simulink model "LineFollowerSim"  (R2021b)
settings: Solver=FixedStepDiscrete  StartTime=0.0  StopTime=10  FixedStep=0.1  RelTol=1e-3  EnableMultiTasking=on
libraries: arduinolib x8, arduinosensorlib x1
settings Model: ExtModeTrigDuration=2  Creator=arjun  LastModifiedBy=arjun
settings SolverCC: AlgebraicLoopSolver=TrustRegion  AutoInsertRateTranBlk=on
settings DataIOCC: LimitDataPoints=on
settings OptimizationCC: EnhancedBackFolding=on  PassReuseOutputArgsAs=Individual arguments  ZeroExternalMemoryAtStartup=off  ZeroInternalMemoryAtStartup=off  MaxStackSize=64  OptimizeBlockOrder=speed  DifferentSizesBufferReuse=on  OptimizationCustomize=off  EfficientTunableParamExpr=on
settings DebuggingCC: ParameterTunabilityLossMsg=error  AllowSymbolicDim=off  SFUnexpectedBacktrackingDiag=warning  SFNoUnconditionalDefaultTransitionDiag=warning  SFExecutionAtInitializationDiag=none  ArithmeticOperatorsInVariantConditions=warning
settings HardwareCC: ProdBitPerInt=16  ProdBitPerPointer=16  ProdBitPerSizeT=16  ProdBitPerPtrDiffT=16  ProdLargestAtomicFloat=None  ProdWordSize=8  ProdHWDeviceType=Atmel->AVR
settings SFSimCC: SimUseLocalCustomCode=off  MATLABDynamicMemAlloc=off  CustomCodeUndefinedFunction=UseInterfaceOnly
settings RTWCC: Description=Embedded Coder  SystemTargetFile=ert.tlc  HardwareBoard=Arduino Uno  TemplateMakefile=ert_default_tmf  RTWUseLocalCustomCode=off  Toolchain=Arduino AVR  BuildConfiguration=Faster Runs
settings CodeAppCC: ForceParamTrailComments=on  IgnoreCustomStorageClasses=off  OperatorAnnotations=on  SimulinkDataObjDesc=on  SFDataObjDesc=on  InsertBlockDesc=on
settings ERTTargetCC: SupportContinuousTime=on  SupportVariableSizeSignals=on  ExtModeTransport=3  ExtModeStaticAlloc=on  ExtModeStaticAllocSize=250  ExtModeMexFile=ext_xcp  ExtModeIntrfLevel=Level2 - Open
settings ConfigComp: CovMetricSettings=dw  CovSaveCumulativeToWorkspaceVar=on  CovSaveSingleToWorkspaceVar=on  CovExternalEMLEnable=off  CovSFcnEnable=off

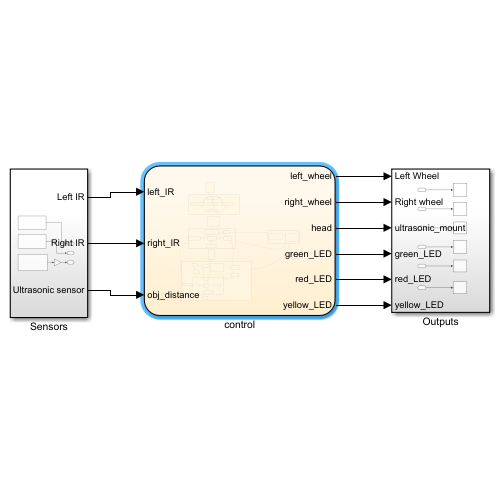
[thumbnail: Simulink's stored preview of the top-level diagram]
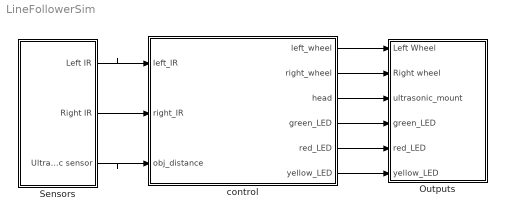
== system LineFollowerSim ==
  Outputs : Subsystem
  Sensors : Subsystem
  control : Stateflow chart  TreatAsAtomicUnit=on
  wires:
  Sensors/1(Left IR) -> control/1(left_IR)
  Sensors/2(Right IR) -> control/2(right_IR)
  Sensors/3(Ultrasonic sensor) -> control/3(obj_distance)
  control/1(left_wheel) -> Outputs/1(Left Wheel)
  control/2(right_wheel) -> Outputs/2(Right wheel)
  control/3(head) -> Outputs/3(ultrasonic_mount)
  control/4(green_LED) -> Outputs/4(green_LED)
  control/5(red_LED) -> Outputs/5(red_LED)
  control/6(yellow_LED) -> Outputs/6(yellow_LED)

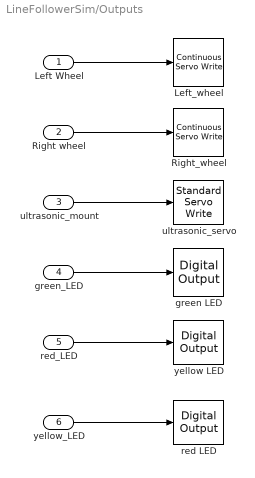
== system LineFollowerSim/Outputs ==
  Left Wheel : Inport
  Right wheel : Inport  Port=2
  ultrasonic_mount : Inport  Port=3
  green_LED : Inport  Port=4
  red_LED : Inport  Port=5
  yellow_LED : Inport  Port=6
  Left_wheel : arduinolib/Continuous Servo Write  pinNumber=11  ServoIndex=0  blockPlatform=ARDUINO
      settings: SourceProductBaseCode=ARDUINO
  Right_wheel : arduinolib/Continuous Servo Write  pinNumber=10  ServoIndex=1  blockPlatform=ARDUINO
      settings: SourceProductBaseCode=ARDUINO
  green LED : arduinolib/Digital Output  pinNumber=4  Direction=output  blockPlatform=arduino
  red LED : arduinolib/Digital Output  pinNumber=6  Direction=output  blockPlatform=arduino
  ultrasonic_servo : arduinolib/Standard Servo Write  pinNumber=9  ServoIndex=2  blockPlatform=ARDUINO
  yellow LED : arduinolib/Digital Output  pinNumber=5  Direction=output  blockPlatform=arduino
  wires:
  ultrasonic_mount/1 -> ultrasonic_servo/1
  Right wheel/1 -> Right_wheel/1
  Left Wheel/1 -> Left_wheel/1
  green_LED/1 -> green LED/1
  red_LED/1 -> yellow LED/1
  yellow_LED/1 -> red LED/1

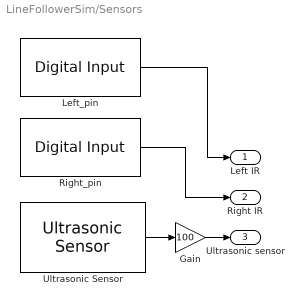
== system LineFollowerSim/Sensors ==
  Gain : Gain  Gain=100
  Left_pin : arduinolib/Digital Input  pinNumber=7  mode=Default  Direction=input  SampleTime=0.1  blockPlatform=arduino
  Right_pin : arduinolib/Digital Input  pinNumber=8  mode=Default  Direction=input  SampleTime=0.1  blockPlatform=arduino
  Ultrasonic Sensor : arduinosensorlib/Ultrasonic Sensor  NumSignalPins=2  TrigPin=5  EchoPin=6  SignalPin=3  SampleTime_=0.1  blockPlatform=ARDUINO
      settings: SourceProductBaseCode=ARDUINO
  Left IR : Outport
  Right IR : Outport  Port=2
  Ultrasonic sensor : Outport  Port=3
  wires:
  Right_pin/1 -> Right IR/1
  Left_pin/1 -> Left IR/1
  Ultrasonic Sensor/1 -> Gain/1
  Gain/1 -> Ultrasonic sensor/1

== stateflow chart LineFollowerSim/control ==
  state Initialize
    entry:
    intersection=0;
    right_IR;
    left_IR;
    right_wheel;
    left_wheel;
    left_adjustment=0;
    right_adjustment=0;
    drive_delay=50;
    adjust_delay=100;
    turn_delay=2000;
    reverse_delay=1800;
    green_LED=0;
    yellow_LED=0;
    red_LED=0;
  state Home_to_start
    state Find_Start
      entry:
      right_wheel=0;
      left_wheel=0;
    state Adjust_left
      entry:
      right_wheel=4;
      left_wheel=0;
    state Follow_Line
      entry:
      right_wheel=4;
      left_wheel=-4;
    state Adjust_right
      entry:
      right_wheel=0;
      left_wheel=-4;
    state Intersection
      intersection = intersection + 1;
    (default) -> Find_Start
    Find_Start -> Home_to_start.Adjust_right [order 2] : [right_IR==1&&left_IR==0]{right_adjustment = right_adjustment + 1}
    Find_Start -> Home_to_start.Adjust_left [order 3] : [right_IR==0&&left_IR==1]{left_adjustment = left_adjustment + 1}
    Home_to_start.Adjust_right -> Find_Start : after(adjust_delay,msec)
    Home_to_start.Adjust_left -> Find_Start : after(adjust_delay,msec)
    Follow_Line -> Find_Start : after(drive_delay,msec)
    Find_Start -> Follow_Line [order 4] : [right_IR==0&&left_IR==0]
    Find_Start -> Intersection [order 1] : [right_IR==1&&left_IR==1]
    Intersection -> Home_to_start.Adjust_left [order 1] : [intersection==1&&left_adjustment>right_adjustment]
    Intersection -> Home_to_start.Adjust_right [order 2] : [intersection==1&&left_adjustment<right_adjustment]
  state On_i0
    entry:
    red_LED=1; %blink RED
    after(1000,msec);
    red_LED=0;
    intersection=0; %reset
    objects_detected=0;
    right_wheel=4;
    left_wheel=-4;
    obj_distance;
    boolean obj_left=false;
    boolean obj_right=false;
    head;
    max_dist=60;
    min_dist=8;
    boolean main_road=true;
  state Intersection_finder
    state Found_intersection
      entry:
      %blink red LED
      intersection = intersection + 1;
      right_wheel=0;
      left_wheel=0;
    state Blink_red
      entry:
      red_LED=1;
      after(1000,msec);
      red_LED=0;
    state Adjust_left
      entry:
      right_wheel=4;
      left_wheel=0;
    state Find_intersection
      entry:
      right_wheel=0;
      left_wheel=0;
    state Adjust_right
      entry:
      right_wheel=0;
      left_wheel=-4;
    state Follow_line
      entry:
      right_wheel=4;
      left_wheel=-4;
    Found_intersection -> Blink_red [order 1] : [main_road==true]
    Find_intersection -> Found_intersection [order 1] : [left_IR==1&&right_IR==1]
    (default) -> Find_intersection
    Find_intersection -> Intersection_finder.Adjust_right [order 2] : [left_IR==0&&right_IR==1]
    Find_intersection -> Intersection_finder.Adjust_left [order 3] : [left_IR==1&&right_IR==0]
    Intersection_finder.Adjust_right -> Find_intersection : after(adjust_delay,msec)
    Intersection_finder.Adjust_left -> Find_intersection : after(adjust_delay,msec)
    Intersection_finder.Follow_line -> Find_intersection : after(drive_delay,msec)
    Find_intersection -> Intersection_finder.Follow_line [order 4] : [left_IR==0&&right_IR==0]
  state Search_object
    state Sweep_right
      entry:
      head=0;
      obj_right=(obj_distance)&(obj_distance<max_dist)
      after(2000,msec);
      if(obj_right)
      yellow_LED=1;
      after(1000,msec);
      yellow_LED=0;
      end
    state Sweep_left
      entry:
      head=180;
      obj_left=(obj_distance)&(obj_distance<max_dist)
      after(2000,msec);
      if(obj_left)
      yellow_LED=1;
      after(1000,msec);
      yellow_LED=0;
      %blink yellow LED
      end
      exit:
      head=90;
    (default) -> Sweep_right
    Sweep_right -> Sweep_left
  state Celebrator
    entry:
    red_LED=1;
    after(200,msec);
    red_LED=0;
    green_LED=1;
    after(200,msec);
    green_LED=0;
    yellow_LED=1;
    after(200,msec);
    yellow_LED=0;
    green_LED=1;
    after(200,msec);
    green_LED=0;
    red_LED=1;
    after(200,msec);
    red_LED=0;
  state Go_to_object
    state spot_turn
      entry:
      main_road=false;
      %dummy
    state Turn_to_main_road
      entry:
      if((obj_right==true)&&(obj_left==false))
      right_wheel=0;
      left_wheel=-20;
      else
      right_wheel=20;
      left_wheel=0;
      end
      obj_left=false;
      obj_right=false;
      main_road=true;
    state turn_right
      entry:
      right_wheel=0;
      left_wheel=-20;
    state At_intersection
      %dummy
    state turn_left
      entry:
      right_wheel=20;
      left_wheel=0;
    state clear_left
      entry:
      right_wheel=5;
      left_wheel=-5;
    state approach_object
      state Follow_line
        entry:
        right_wheel=4;
        left_wheel=-4;
      state Adjust_left
        entry:
        right_wheel=4;
        left_wheel=0;
      state Finder
        entry:
        right_wheel=0;
        left_wheel=0;
      state Adjust_right
        entry:
        right_wheel=0;
        left_wheel=-4;
      state Obj_found
        entry:
        right_wheel=0;
        left_wheel=0;
        objects_detected = objects_detected + 1;
        %blink green LED
      Go_to_object.approach_object.Follow_line -> Finder : after(drive_delay,msec)
      Finder -> Go_to_object.approach_object.Follow_line [order 2] : [left_IR==0&&right_IR==0]
      (default) -> Finder
      Finder -> Go_to_object.approach_object.Adjust_right [order 3] : [left_IR==0&&right_IR==1]
      Finder -> Go_to_object.approach_object.Adjust_left [order 4] : [left_IR==1&&right_IR==0]
      Go_to_object.approach_object.Adjust_right -> Finder : after(adjust_delay,msec)
      Go_to_object.approach_object.Adjust_left -> Finder : after(adjust_delay,msec)
      Finder -> Obj_found [order 1] : [obj_distance<=min_dist]
    state goto_intersection
    state turn_around
      entry:
      right_wheel=-20;
      left_wheel=-20;
      %essentially turning right twice
    state Blink_green
      entry:
      green_LED=1;
      after(1000,msec);
      green_LED=0;
    (default) -> spot_turn
    spot_turn -> turn_right [order 2] : [(obj_right==true)]
    spot_turn -> turn_left [order 1] : [(obj_right==false)&&(obj_left==true)]
    At_intersection -> Turn_to_main_road [order 2]
    turn_right -> approach_object : after(turn_delay,msec)
    At_intersection -> clear_left [order 1] : [(obj_right==true)&&(obj_left==true)]
    Turn_to_main_road -> approach_object [order 2] : [intersection==5&&objects_detected==4]
    turn_left -> approach_object : after(turn_delay,msec)
    clear_left -> approach_object : after(500,msec){obj_right=false} %to pass the intersection
    turn_around -> goto_intersection : after(reverse_delay,msec)
    Obj_found -> Blink_green
    Blink_green -> turn_around
  (default) -> Initialize
  Initialize -> Home_to_start
  Home_to_start -> On_i0 : [intersection==2]{right_wheel=0;left_wheel=0}
  On_i0 -> Intersection_finder : after(500,msec)%to pass i0
  Blink_red -> Search_object
  Found_intersection -> At_intersection [order 2]
  Sweep_left -> Intersection_finder [order 1] : [(obj_right==false)&&(obj_left==false)]
  Sweep_left -> Go_to_object [order 2]
  goto_intersection -> Intersection_finder
  approach_object -> Celebrator : [objects_detected==5&&main_road==true]
  Turn_to_main_road -> Celebrator [order 1] : [objects_detected==5]
  data: left_IR input; right_IR input; objects_detected local; intersection local; left_wheel output; right_wheel output; left_adjustment local; right_adjustment local; obj_distance input; head output; obj_right local; max_dist local; obj_left local; min_dist local; main_road local; adjust_delay constant double; drive_delay constant double; reverse_delay constant double; turn_delay constant double; green_LED output; red_LED output; yellow_LED output
